simulink model "foc"  (R2016a)
settings: Solver=ode1  StartTime=0.0  StopTime=2  FixedStep=10e-6  RelTol=1e-8
libraries: powerlib x29, simulink x2, simulink_extras x1, powerlib_meascontrol x1
settings Model: Creator=mtech  LastModifiedBy=Dharma
settings DebuggingCC: MaxConsecutiveZCsMsg=none

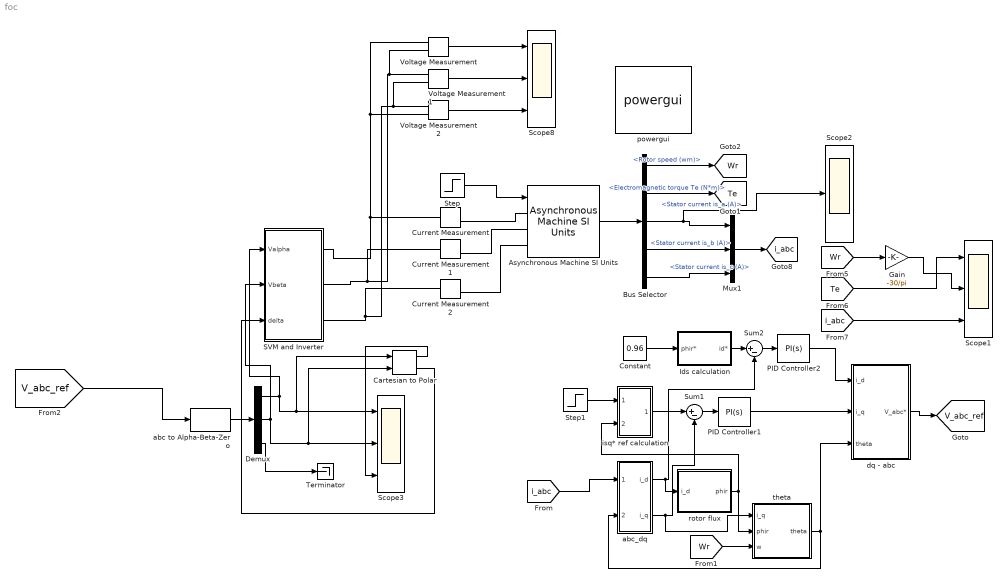
== system foc ==
  Asynchronous Machine SI Units : powerlib/Machines/Asynchronous Machine SI Units  RotorType=Squirrel-cage  PresetModel="15:  5.4 HP (4KW)   400 V  50Hz 1430 RPM"  MechanicalLoad=Torque Tm  ShowDetailedParameters=on  ReferenceFrame=Stationary  Units=SI  MeasurementBus=off  NominalParameters=[4000 400 50]  Stator=[1.405 0.005839]  Rotor=[1.395 0.005839]  Cage1=[0.4155 0.002066]  Cage2=[0.4168 0.0003495]  Lm=0.1722  Mechanical=[0.0131 0.002985 2]  PolePairs=2  InitialConditions=[1 0 0 0 0 0 0 0]  SimulateSaturation=off  Saturation=[14.03593122, 27.81365428, 53.79336849, 72.68890987, 97.98006896, 148.6815601, 215.7428561, 302.9841135, 428.7778367 ; 230, 322, 414, 460, 506, 552, 598, 644, 690]  LoadFlowParameters=1492000  TsPowergui=0  TsBlock=-1  IterativeModel=Trapezoidal non iterative  IterativeDiscreteModel=Trapezoidal non iterative  Pmec=1.492e+006
  Bus Selector : BusSelector  OutputSignals=Mechanical.Rotor speed (wm),Mechanical.Electromagnetic torque Te (N*m),Stator measurements.Stator current is_a (A),Stator measurements.Stator current is_b (A),Stator measurements.Stator current is_c (A)
  Cartesian to Polar : simulink_extras/Transformations/Cartesian to Polar
  Constant : Constant  Value=0.96
  Current Measurement : powerlib/Measurements/Current Measurement  PhasorSimulation=off  OutputType=Complex  PSBequivalent=0
  Current Measurement1 : powerlib/Measurements/Current Measurement  PhasorSimulation=off  OutputType=Complex  PSBequivalent=0
  Current Measurement2 : powerlib/Measurements/Current Measurement  PhasorSimulation=off  OutputType=Complex  PSBequivalent=0
  Demux : Demux  Outputs=3
  Gain : Gain  Gain=-30/pi
  Ids calculation : Subsystem
  Mux1 : Mux  Inputs=3
  PID Controller1 : simulink/Continuous/PID Controller  Controller=PI  TimeDomain=Continuous-time  SampleTime=-1  IntegratorMethod=Forward Euler  FilterMethod=Forward Euler  Form=Parallel  UseFilter=on  ControllerParametersSource=internal  P=100  I=0  D=0  N=100  InitialConditionSource=internal  InitialConditionForIntegrator=0  InitialConditionForFilter=0  ExternalReset=none  LimitOutput=off  UpperSaturationLimit=inf  LowerSaturationLimit=-inf  LinearizeAsGain=on  AntiWindupMode=none  Kb=1  TrackingMode=off  Kt=1  PParamMin=[]  PParamMax=[]  IParamMin=[]  IParamMax=[]  DParamMin=[]  DParamMax=[]  NParamMin=[]  NParamMax=[]  KbParamMin=[]  KbParamMax=[]  KtParamMin=[]  KtParamMax=[]  POutMin=[]  POutMax=[]  IOutMin=[]  IOutMax=[]  DOutMin=[]  DOutMax=[]  NOutMin=[]  NOutMax=[]  KbOutMin=[]  KbOutMax=[]  KtOutMin=[]  KtOutMax=[]  IntegratorOutMin=[]  IntegratorOutMax=[]  FilterOutMin=[]  FilterOutMax=[]  SumOutMin=[]  SumOutMax=[]  SumI1OutMin=[]  SumI1OutMax=[]  SumI2OutMin=[]  SumI2OutMax=[]  SumI3OutMin=[]  SumI3OutMax=[]  SumDOutMin=[]  SumDOutMax=[]  SaturationOutMin=[]  SaturationOutMax=[]  IntegratorContinuousStateAttributes=''  IntegratorStateMustResolveToSignalObject=off  IntegratorRTWStateStorageClass=Auto  FilterContinuousStateAttributes=''  FilterStateMustResolveToSignalObject=off  FilterRTWStateStorageClass=Auto  DifferentiatorICPrevScaledInput=0  DifferentiatorOutMin=[]  DifferentiatorOutMax=[]
  PID Controller2 : simulink/Continuous/PID Controller  Controller=PI  TimeDomain=Continuous-time  SampleTime=-1  IntegratorMethod=Forward Euler  FilterMethod=Forward Euler  Form=Parallel  UseFilter=on  ControllerParametersSource=internal  P=100  I=0  D=0  N=100  InitialConditionSource=internal  InitialConditionForIntegrator=0  InitialConditionForFilter=0  ExternalReset=none  LimitOutput=off  UpperSaturationLimit=inf  LowerSaturationLimit=-inf  LinearizeAsGain=on  AntiWindupMode=none  Kb=1  TrackingMode=off  Kt=1  PParamMin=[]  PParamMax=[]  IParamMin=[]  IParamMax=[]  DParamMin=[]  DParamMax=[]  NParamMin=[]  NParamMax=[]  KbParamMin=[]  KbParamMax=[]  KtParamMin=[]  KtParamMax=[]  POutMin=[]  POutMax=[]  IOutMin=[]  IOutMax=[]  DOutMin=[]  DOutMax=[]  NOutMin=[]  NOutMax=[]  KbOutMin=[]  KbOutMax=[]  KtOutMin=[]  KtOutMax=[]  IntegratorOutMin=[]  IntegratorOutMax=[]  FilterOutMin=[]  FilterOutMax=[]  SumOutMin=[]  SumOutMax=[]  SumI1OutMin=[]  SumI1OutMax=[]  SumI2OutMin=[]  SumI2OutMax=[]  SumI3OutMin=[]  SumI3OutMax=[]  SumDOutMin=[]  SumDOutMax=[]  SaturationOutMin=[]  SaturationOutMax=[]  IntegratorContinuousStateAttributes=''  IntegratorStateMustResolveToSignalObject=off  IntegratorRTWStateStorageClass=Auto  FilterContinuousStateAttributes=''  FilterStateMustResolveToSignalObject=off  FilterRTWStateStorageClass=Auto  DifferentiatorICPrevScaledInput=0  DifferentiatorOutMin=[]  DifferentiatorOutMax=[]
  SVM and Inverter : Subsystem
  Scope1 : Scope  NumInputPorts=3
  Scope2 : Scope
  Scope3 : Scope  NumInputPorts=3
  Scope8 : Scope  NumInputPorts=3
  Step : Step  Before=10  After=20  SampleTime=0
  Step1 : Step  Before=10  After=20  SampleTime=0
  Sum1 : Sum  Inputs=|+-
  Sum2 : Sum  Inputs=|+-
  Terminator : Terminator
  Voltage Measurement : powerlib/Measurements/Voltage Measurement  PhasorSimulation=off  OutputType=Complex  PSBequivalent=0
  Voltage Measurement1 : powerlib/Measurements/Voltage Measurement  PhasorSimulation=off  OutputType=Complex  PSBequivalent=0
  Voltage Measurement2 : powerlib/Measurements/Voltage Measurement  PhasorSimulation=off  OutputType=Complex  PSBequivalent=0
  abc to Alpha-Beta-Zero : powerlib_meascontrol/Transformations/abc to Alpha-Beta-Zero
  abc_dq : Subsystem
  dq - abc : Subsystem
  isq* ref calculation : Subsystem
  powergui : powerlib/powergui  Priority=1  SimulationMode=Discrete  SolverType=Tustin/Backward Euler (TBE)  SampleTime=10e-6  frequency=60  SPID=off  DisableSnubberDevices=off  DisableRonSwitches=off  DisableVfSwitches=off  SwTol=0  DisplayEquations=off  Interpol=off  ExternalGateDelay=off  methode=off  Ts=10  FunctionMessages=off  echomessages=off  HookPort=off  EnableUseOfTLC=off  x0status=blocks  frequencyindice=0  Pbase=100e6  ErrMax=1e-4  Iterations=50  UnitsV=kV  UnitsW=MW  buscounter=0  RestoreLinks=warning  ResistiveCurrentMeasurement=off  Frange=[0:2:500]  Ylog=off  Xlog=on  ShowGrid=off  save=off  variable=ZData  structure=ia  ZoomFFT=off  StartTime=0.35  cycles=1  DisplayStyle=1  fundamental=43  FreqAxis=on  MaxFrequency=1000  frequencyindicesteady=1  RmsSteady=1  display=off
  rotor flux : Subsystem
  theta : Subsystem
  tag scope: Te=global, V_abc_ref=global, Wr=global, i_abc=global
  wires:
  Voltage Measurement/1 -> Scope8/1
  Voltage Measurement1/1 -> Scope8/2
  Voltage Measurement2/1 -> Scope8/3
  Asynchronous Machine SI Units/1 -> Bus Selector/1
  Bus Selector/1 -> [Wr]  "<Rotor speed (wm)>"
  Bus Selector/2 -> [Te]  "<Electromagnetic torque Te (N*m)>"
  Bus Selector/3 -> Scope2/1, Mux1/1  "<Stator current is_a (A)>"
  Bus Selector/4 -> Mux1/2  "<Stator current is_b (A)>"
  Bus Selector/5 -> Mux1/3  "<Stator current is_c (A)>"
  Mux1/1 -> [i_abc]
  [V_abc_ref] -> abc to Alpha-Beta-Zero/1
  abc to Alpha-Beta-Zero/1 -> Demux/1
  Demux/1 -> SVM and Inverter/1(Valpha), Cartesian to Polar/1, Scope3/1
  Demux/2 -> SVM and Inverter/2(Vbeta), Cartesian to Polar/2, Scope3/2
  Cartesian to Polar/2 -> SVM and Inverter/3(delta)
  Cartesian to Polar/1 -> Scope3/3
  Demux/3 -> Terminator/1
  Step/1 -> Asynchronous Machine SI Units/1
  [Wr] -> Gain/1
  [i_abc] -> Scope1/3
  [i_abc] -> abc_dq/1(i_abc)
  abc_dq/2(i_q) -> Sum1/2, theta/1(i_q)
  abc_dq/1(i_d) -> Sum2/2, rotor flux/1(i_d)
  rotor flux/1(phir) -> theta/2(phir), isq* ref calculation/2(phir)
  Step1/1 -> isq* ref calculation/1(Te*)
  [Wr] -> theta/3(w)
  Constant/1 -> Ids calculation/1(phir*)
  isq* ref calculation/1(isq*) -> Sum1/1
  Sum1/1 -> PID Controller1/1
  Ids calculation/1(id*) -> Sum2/1
  PID Controller1/1 -> dq - abc/2(i_q)
  Sum2/1 -> PID Controller2/1
  PID Controller2/1 -> dq - abc/1(i_d)
  dq - abc/1(V_abc*) -> [V_abc_ref]
  theta/1(theta) -> abc_dq/2(theta), dq - abc/3(theta)
  [Te] -> Scope1/1
  Gain/1 -> Scope1/2
  connections:
  Current Measurement/LConn1 -- SVM and Inverter/RConn1 -- Voltage Measurement2/LConn2 -- Voltage Measurement/LConn1
  Current Measurement1/LConn1 -- SVM and Inverter/RConn2 -- Voltage Measurement/LConn2 -- Voltage Measurement1/LConn1
  Current Measurement2/LConn1 -- SVM and Inverter/RConn3 -- Voltage Measurement1/LConn2 -- Voltage Measurement2/LConn1
  Current Measurement2/RConn1 -- Asynchronous Machine SI Units/LConn3
  Current Measurement1/RConn1 -- Asynchronous Machine SI Units/LConn2
  Current Measurement/RConn1 -- Asynchronous Machine SI Units/LConn1

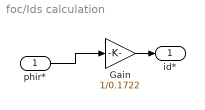
== system foc/Ids calculation ==
  phir* : Inport
  Gain : Gain  Gain=1/0.1722
  id* : Outport
  wires:
  Gain/1 -> id*/1
  phir*/1 -> Gain/1

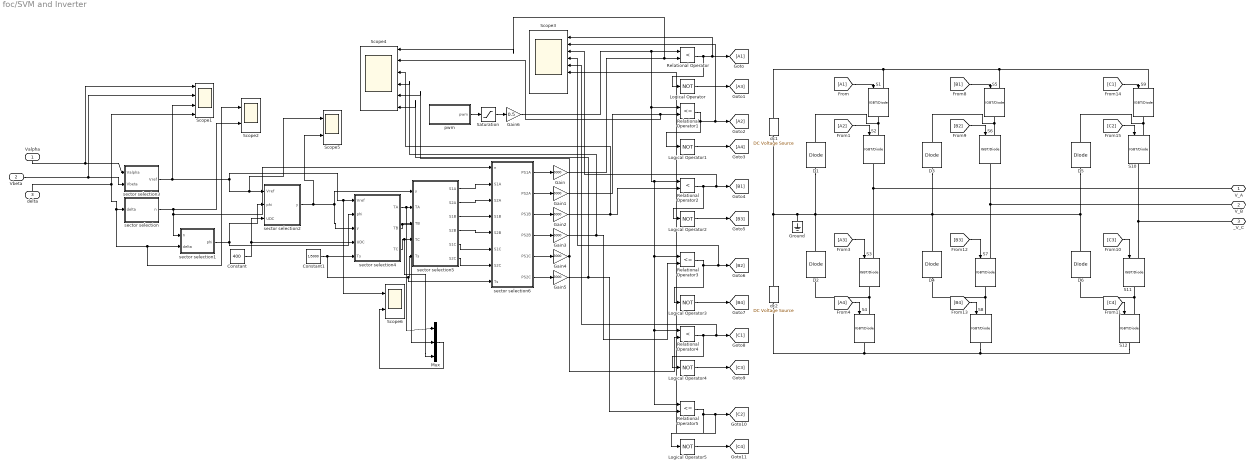
== system foc/SVM and Inverter ==
  Valpha : Inport
  Vbeta : Inport  Port=2
  delta : Inport  Port=3
  Constant : Constant  Value=400
  Constant1 : Constant  Value=1/5000
  D{1..6} (6 alike) : powerlib/Power Electronics/Diode  Ron=0.001  Lon=0  Vf=0.8  IC=0  UseSnubber=off  Rs=500  Cs=250e-9  Measurements=off
  Gain{,1..5} (6 alike) : Gain  Gain=5000
  Gain6 : Gain  Gain=0.5
  Ground : powerlib/Elements/Ground  LConnTagsString=a
  Logical Operator{,1..5} (6 alike) : Logic  Operator=NOT  AllPortsSameDT=off  OutDataTypeStr=boolean
  Mux : Mux  Inputs=3
  Relational Operator : RelationalOperator  Operator=<  OutDataTypeStr=boolean
  Relational Operator1 : RelationalOperator  Operator=<=  OutDataTypeStr=boolean
  Relational Operator2 : RelationalOperator  Operator=<  OutDataTypeStr=boolean
  Relational Operator3 : RelationalOperator  Operator=<=  OutDataTypeStr=boolean
  Relational Operator4 : RelationalOperator  Operator=<  OutDataTypeStr=boolean
  Relational Operator5 : RelationalOperator  Operator=<=  OutDataTypeStr=boolean
  S{1..12} (12 alike) : powerlib/Power Electronics/IGBT//Diode  Ron=1e-3  Rs=1e5  Cs=inf  Measurements=off
  Saturation : Saturate  UpperLimit=1  LowerLimit=0
  Scope1 : Scope  NumInputPorts=4
  Scope2 : Scope  NumInputPorts=2
  Scope3 : Scope  NumInputPorts=8
  Scope4 : Scope  NumInputPorts=6
  Scope5 : Scope  NumInputPorts=2
  Scope6 : Scope  NumInputPorts=2
  dc1 : powerlib/Electrical Sources/DC Voltage Source  Amplitude=200  Measurements=None
  dc2 : powerlib/Electrical Sources/DC Voltage Source  Amplitude=200  Measurements=None
  pwm : Subsystem
  sector selection : MATLAB Function  TreatAsAtomicUnit=on
  sector selection1 : MATLAB Function  TreatAsAtomicUnit=on
  sector selection2 : MATLAB Function  TreatAsAtomicUnit=on
  sector selection3 : MATLAB Function  TreatAsAtomicUnit=on
  sector selection4 : MATLAB Function  TreatAsAtomicUnit=on
  sector selection5 : MATLAB Function  TreatAsAtomicUnit=on
  sector selection6 : MATLAB Function  TreatAsAtomicUnit=on
  V_A : PMIOPort  Port=1  Side=Right
  V_B : PMIOPort  Port=2  Side=Right
  _V_C : PMIOPort  Port=3  Side=Right
  wires:
  sector selection3/1(Vref) -> Scope1/3, Scope5/1, sector selection2/1(Vref), Scope6/1, sector selection4/1(Vref)
  sector selection5/4(S2B) -> sector selection6/5(S2B)
  sector selection5/5(S1C) -> sector selection6/6(S1C)
  sector selection6/4(PS2B) -> Gain3/1
  sector selection5/6(S2C) -> sector selection6/7(S2C)
  sector selection4/2(TB) -> Mux/2, sector selection5/3(TB)
  sector selection1/1(phi) -> sector selection2/2(phi), sector selection4/2(phi)
  sector selection5/1(S1A) -> sector selection6/2(S1A)
  sector selection6/2(PS2A) -> Gain1/1
  sector selection2/1(y) -> Scope5/2, sector selection4/3(y), sector selection5/1(y)
  sector selection5/2(S2A) -> sector selection6/3(S2A)
  sector selection4/1(TA) -> Mux/1, sector selection5/2(TA)
  sector selection4/3(TC) -> Mux/3, sector selection5/4(TC)
  sector selection6/5(PS1C) -> Gain4/1
  Vbeta/1 -> Scope1/2, sector selection3/2(Vbeta)
  Constant1/1 -> sector selection6/8(Ts), sector selection5/5(Ts), sector selection4/5(Ts)
  sector selection5/3(S1B) -> sector selection6/4(S1B)
  Constant/1 -> sector selection2/3(UDC), sector selection4/4(UDC)
  Logical Operator2/1 -> [B3]
  sector selection6/3(PS1B) -> Gain2/1
  Logical Operator4/1 -> [C3]
  Gain6/1 -> Relational Operator5/1, Relational Operator4/1, Relational Operator3/1, Relational Operator2/1, Relational Operator1/1, Relational Operator/1
  Relational Operator/1 -> Scope3/1, [A1], Logical Operator/1
  Logical Operator/1 -> [A3]
  Gain3/1 -> Scope4/4, Relational Operator3/2
  Logical Operator3/1 -> [B4]
  Relational Operator3/1 -> Scope3/4, [B2], Logical Operator3/1
  Relational Operator2/1 -> Logical Operator2/1, Scope3/3, [B1]
  Gain/1 -> Scope4/1, Relational Operator/2
  sector selection6/1(PS1A) -> Gain/1
  Relational Operator1/1 -> Scope3/2, [A2], Logical Operator1/1
  pwm/1("pwm ") -> Saturation/1
  Logical Operator1/1 -> [A4]
  Logical Operator5/1 -> [C4]
  Gain1/1 -> Scope4/2, Relational Operator1/2
  Relational Operator5/1 -> Logical Operator5/1, Scope3/6, [C2]
  Saturation/1 -> Gain6/1
  Gain5/1 -> Scope4/6, Relational Operator5/2
  sector selection/1(n) -> Scope2/2, sector selection1/1(n), sector selection6/1(n)
  Gain4/1 -> Relational Operator4/2, Scope4/5
  delta/1 -> Scope1/4, sector selection/1(delta), Scope2/1, sector selection1/2(delta)
  Gain2/1 -> Scope4/3, Relational Operator2/2
  sector selection6/6(PS2C) -> Gain5/1
  Relational Operator4/1 -> Logical Operator4/1, Scope3/5, [C1]
  Valpha/1 -> Scope1/1, sector selection3/1(Valpha)
  Mux/1 -> Scope6/2
  [A4] -> S4/1
  [A2] -> S2/1
  [B1] -> S5/1
  [C1] -> S9/1
  [C2] -> S10/1
  [B2] -> S6/1
  [C3] -> S11/1
  [B3] -> S7/1
  [A3] -> S3/1
  [B4] -> S8/1
  [A1] -> S1/1
  [C4] -> S12/1
  connections:
  S8/RConn1 -- S12/RConn1 -- S4/RConn1 -- dc2/LConn1
  S9/LConn1 -- S5/LConn1 -- dc1/RConn1 -- S1/LConn1
  D4/LConn1 -- S8/LConn1 -- S7/RConn1
  S10/LConn1 -- D5/RConn1 -- S9/RConn1
  D3/RConn1 -- S6/LConn1 -- S5/RConn1
  S2/LConn1 -- D1/RConn1 -- S1/RConn1
  dc1/LConn1 -- dc2/RConn1 -- Ground/LConn1 -- D1/LConn1 -- D2/RConn1 -- D3/LConn1 -- D4/RConn1 -- D5/LConn1 -- D6/RConn1
  S2/RConn1 -- V_A/RConn1 -- S3/LConn1
  D6/LConn1 -- S12/LConn1 -- S11/RConn1
  S6/RConn1 -- V_B/RConn1 -- S7/LConn1
  S10/RConn1 -- _V_C/RConn1 -- S11/LConn1
  D2/LConn1 -- S4/LConn1 -- S3/RConn1

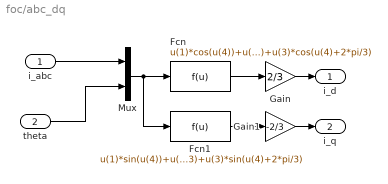
== system foc/abc_dq ==
  i_abc : Inport
  theta : Inport  Port=2
  Fcn : Fcn  Expr=u(1)*cos(u(4))+u(2)*cos(u(4)-2*pi/3)+u(3)*cos(u(4)+2*pi/3)
  Fcn1 : Fcn  Expr=u(1)*sin(u(4))+u(2)*sin(u(4)-2*pi/3)+u(3)*sin(u(4)+2*pi/3)
  Gain : Gain  Gain=2/3
  Gain1 : Gain  Gain=-2/3
  Mux : Mux  Inputs=2
  i_d : Outport
  i_q : Outport  Port=2
  wires:
  Fcn1/1 -> Gain1/1
  Gain/1 -> i_d/1
  Gain1/1 -> i_q/1
  Fcn/1 -> Gain/1
  theta/1 -> Mux/2
  Mux/1 -> Fcn1/1, Fcn/1
  i_abc/1 -> Mux/1

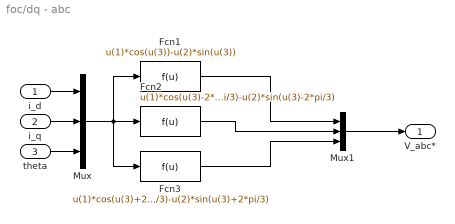
== system foc/dq - abc ==
  i_d : Inport
  i_q : Inport  Port=2
  theta : Inport  Port=3
  Fcn1 : Fcn  Expr=u(1)*cos(u(3))-u(2)*sin(u(3))
  Fcn2 : Fcn  Expr=u(1)*cos(u(3)-2*pi/3)-u(2)*sin(u(3)-2*pi/3)
  Fcn3 : Fcn  Expr=u(1)*cos(u(3)+2*pi/3)-u(2)*sin(u(3)+2*pi/3)
  Mux : Mux  Inputs=3
  Mux1 : Mux  Inputs=3
  V_abc* : Outport
  wires:
  i_q/1 -> Mux/2
  i_d/1 -> Mux/1
  Mux/1 -> Fcn3/1, Fcn2/1, Fcn1/1
  theta/1 -> Mux/3
  Fcn3/1 -> Mux1/3
  Fcn1/1 -> Mux1/1
  Fcn2/1 -> Mux1/2
  Mux1/1 -> V_abc*/1

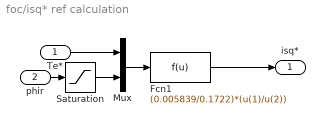
== system foc/isq* ref calculation ==
  Te* : Inport
  phir : Inport  Port=2
  Fcn1 : Fcn  Expr=(0.005839/0.1722)*(u(1)/u(2))
  Mux : Mux  Inputs=2
  Saturation : Saturate  UpperLimit=inf  LowerLimit=1e-3
  isq* : Outport
  wires:
  Mux/1 -> Fcn1/1
  Fcn1/1 -> isq*/1
  phir/1 -> Saturation/1
  Saturation/1 -> Mux/2
  Te*/1 -> Mux/1

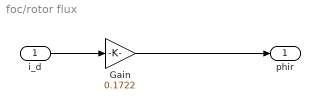
== system foc/rotor flux ==
  i_d : Inport
  Gain : Gain  Gain=0.1722
  phir : Outport
  wires:
  i_d/1 -> Gain/1
  Gain/1 -> phir/1

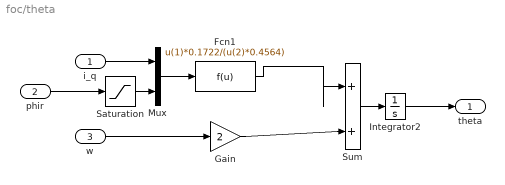
== system foc/theta ==
  i_q : Inport
  phir : Inport  Port=2
  w : Inport  Port=3
  Fcn1 : Fcn  Expr=u(1)*0.1722/(u(2)*0.4564)
  Gain : Gain  Gain=2
  Integrator2 : Integrator
  Mux : Mux  Inputs=2
  Saturation : Saturate  UpperLimit=inf  LowerLimit=1e-3
  Sum : Sum  Inputs=|++
  theta : Outport
  wires:
  phir/1 -> Saturation/1
  Gain/1 -> Sum/2
  i_q/1 -> Mux/1
  w/1 -> Gain/1
  Mux/1 -> Fcn1/1
  Sum/1 -> Integrator2/1
  Saturation/1 -> Mux/2
  Fcn1/1 -> Sum/1
  Integrator2/1 -> theta/1

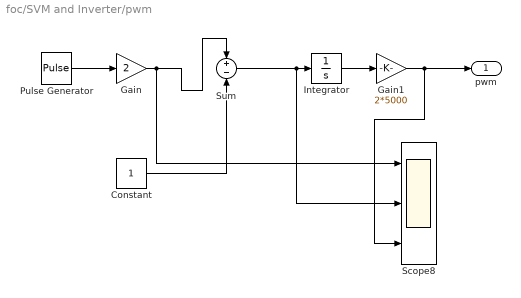
== system foc/SVM and Inverter/pwm ==
  Constant : Constant
  Gain : Gain  Gain=2
  Gain1 : Gain  Gain=2*5000
  Integrator : Integrator
  Pulse Generator : DiscretePulseGenerator  PulseType=Time based  Period=1/5000  PulseWidth=50
  Scope8 : Scope  NumInputPorts=3
  Sum : Sum  Inputs=+-
  "pwm " : Outport
  wires:
  Sum/1 -> Scope8/2, Integrator/1
  Pulse Generator/1 -> Gain/1
  Integrator/1 -> Gain1/1
  Gain/1 -> Scope8/1, Sum/1
  Constant/1 -> Sum/2
  Gain1/1 -> Scope8/3, "pwm "/1

== matlab function foc/SVM and Inverter/sector selection4 ==
  data: Vref input; phi input; y input; UDC input; TA output; Ts input; TB output; TC output
function [TA,TB,TC] =fcn(Vref,phi,y,UDC,Ts)
TA=0;
TB=0;
TC=0;
m=Vref/(2/3*UDC);
k=2/sqrt(3)*m*Ts;

if(y==1)
    TA=2*k*sin(pi/3-phi);
    TB=Ts-2*k*sin(pi/3+phi);
    TC=2*k*sin(phi);
end
if(y==2)
    TC=Ts-2*k*sin(pi/3-phi);
    TB=2*k*sin(pi/3+phi)-Ts;
    TA=Ts-2*k*sin(phi);
end
if(y==3)
    TB=2*k*sin(pi/3-phi);
    TC=2*Ts-2*k*sin(pi/3+phi);
    TA=2*k*sin(phi)-Ts;
end
if(y==4)
    TA=2*Ts-2*k*sin(pi/3+phi);
    TC=2*k*sin(pi/3-phi)-Ts;
    TB=2*k*sin(phi);
end

== matlab function foc/SVM and Inverter/sector selection5 ==
  data: y input; TA input; TB input; S1A output; TC input; Ts input; S2A output; S1B output; S2B output; S1C output; S2C output
function [S1A,S2A,S1B,S2B,S1C,S2C] =fcn(y,TA,TB,TC,Ts)
S1A=0;
S2A=0;
S1B=0;
S2B=0;
S1C=0;
S2C=0;
if(y==1)
    S1A=TC/4+TA/4;
    S2A=Ts/2;
    S1B=TC/4;
    S2B=Ts/2-TA/4;
    S1C=0;
    S2C=Ts/2-TA/4-TC/4;
end
if(y==2)
    S1A=TC/4+TA/4+TB/2;
    S2A=Ts/2;
    S1B=TC/4;
    S2B=Ts/2-TA/4;
    S1C=0;
    S2C=TC/4+TA/4;
end
if(y==3)
    S1A=Ts/2-TC/4;
    S2A=Ts/2;
    S1B=TC/4+TA/2;
    S2B=Ts/2;
    S1C=0;
    S2C=TC/4;
end
if(y==4)
    S1A=Ts/2-TA/4;
    S2A=Ts/2;
    S1B=0;
    S2B=TA/4+TB/2;
    S1C=0;
    S2C=TA/4;
end

== matlab function foc/SVM and Inverter/sector selection6 ==
  data: n input; S1A input; S2A input; PS1A output; S1B input; S2B input; S1C input; S2C input; PS2A output; PS1B output; PS2B output; PS1C output; PS2C output; Ts input
function [PS1A,PS2A,PS1B,PS2B,PS1C,PS2C] =fcn(n,S1A,S2A,S1B,S2B,S1C,S2C,Ts)
PS1A=0;
PS2A=0;
PS1B=0;
PS2B=0;
PS1C=0;
PS2C=0;
if(n==1)
    PS1A=S1A;
    PS2A=S2A;
    PS1B=S1B;
    PS2B=S2B;
    PS1C=S1C;
    PS2C=S2C;
end
if(n==3)
    PS1A=S1C;
    PS2A=S2C;
    PS1B=S1A;
    PS2B=S2A;
    PS1C=S1B;
    PS2C=S2B;
end
if(n==5)
    PS1A=S1B;
    PS2A=S2B;
    PS1B=S1C;
    PS2B=S2C;
    PS1C=S1A;
    PS2C=S2A;
end
if(n==2)
    PS1A=Ts/2-S2B;
    PS2A=Ts/2-S1B;
    PS1B=Ts/2-S2C;
    PS2B=Ts/2-S1C;
    PS1C=Ts/2-S2A;
    PS2C=Ts/2-S1A;
end
if(n==4)
    PS1A=Ts/2-S2A;
    PS2A=Ts/2-S1A;
    PS1B=Ts/2-S2B;
    PS2B=Ts/2-S1B;
    PS1C=Ts/2-S2C;
    PS2C=Ts/2-S1C;
end
if(n==6)
    PS1A=Ts/2-S2C;
    PS2A=Ts/2-S1C;
    PS1B=Ts/2-S2A;
    PS2B=Ts/2-S1A;
    PS1C=Ts/2-S2B;
    PS2C=Ts/2-S1B;
end

== matlab function foc/SVM and Inverter/sector selection ==
  data: delta input; n output
function n = fcn(delta)
n=0;
if (delta>=0)&&(delta<pi/3)
    n=1;
end
if (delta>=pi/3)&&(delta<=2*pi/3)
    n=2;
end
if (delta>=2*pi/3)&&(delta<pi)
    n=3;
end
if (delta>=-pi)&&(delta<-2*pi/3)
    n=4;
end
if (delta>=-2*pi/3)&&(delta<-pi/3)
    n=5;
end
if (delta>=-pi/3)&&(delta<0)
    n=6;
end

== matlab function foc/SVM and Inverter/sector selection1 ==
  data: n input; delta input; phi output
function phi = fcn(n,delta)
phi=0;
if(n==1)
    phi=delta;
end
if(n==2)
    phi=delta-pi/3;
end
if(n==3)
    phi=delta-2*pi/3;
end
if(n==4)
    phi=pi+delta;
end
if(n==5)
    phi=2*pi/3+delta;
end
if(n==6)
    phi=pi/3+delta;
end

== matlab function foc/SVM and Inverter/sector selection2 ==
  data: Vref input; phi input; UDC input; y output
function y =fcn(Vref,phi,UDC)
y=0;
m=Vref/(2/3*UDC);
m1=m*2/sqrt(3)*sin(pi/3-phi);
m2=m*2/sqrt(3)*sin(phi);
if (m1<0.5)&&(m2<0.5)&&(m1+m2<0.5)
    y=1;
end
if (m1<0.5)&&(m2<0.5)&&(m1+m2>0.5)
    y=2;
end
if (m1>0.5)
    y=4;
end
if (m2>0.5)
    y=3;
end

== matlab function foc/SVM and Inverter/sector selection3 ==
  data: Valpha input; Vbeta input; Vref output
function Vref = fcn(Valpha,Vbeta)
Vref=sqrt(Valpha^2+Vbeta^2)
